simulink model "tracked_robot_alg_loop_converges"  (R2023a)
settings: Solver=FixedStepDiscrete  StartTime=0.0  StopTime=sim_param.t_end  FixedStep=sim_param.dt  RelTol=1e-3  EnableMultiTasking=on
InitFcn:
  | tracked_robot_param
undefined symbols (not defined in the file or in its folder): DiscIntNeverNeededParam, param, path_param, sim_param
libraries: simulink x2
settings Model: PacingRate=0.002500  Creator=david  LastModifiedBy=mfocchi
settings SolverCC: AutoInsertRateTranBlk=on
settings OptimizationCC: DefaultParameterBehavior=Inlined  UseDivisionForNetSlopeComputation=on  GainParamInheritBuiltInType=on  UseFloatMulNetSlope=on  InlineInvariantSignals=on  PassReuseOutputArgsAs=Individual arguments  ZeroExternalMemoryAtStartup=off  ZeroInternalMemoryAtStartup=off  NoFixptDivByZeroProtection=on  EfficientFloat2IntCast=on  LifeSpan=1  OptimizeBlockOrder=speed  DifferentSizesBufferReuse=on  EfficientTunableParamExpr=on
settings DebuggingCC: ParameterTunabilityLossMsg=error  UnderSpecifiedDimensionMsg=warning
settings HardwareCC: ProdLongLongMode=on
settings ModelReferenceCC: ModelReferenceMinAlgLoopOccurrences=on
settings SFSimCC: MATLABDynamicMemAlloc=off
settings RTWCC: Description=Embedded Coder  SystemTargetFile=ert.tlc  TemplateMakefile=ert_default_tmf  TargetLang=C++
settings CodeAppCC: ForceParamTrailComments=on  IgnoreCustomStorageClasses=off  OperatorAnnotations=on  SimulinkDataObjDesc=on  SFDataObjDesc=on  CustomSymbolStrGlobalVar=rt$N$M  CustomSymbolStrType=$N$M  CustomSymbolStrFcn=$N$M$F  CustomSymbolStrMacro=$N$M  InsertBlockDesc=on
settings ERTTargetCC: TargetLangStandard=C++11 (ISO)  GenerateSampleERTMain=on  IncludeMdlTerminateFcn=off  CombineSignalStateStructs=on  CodeInterfacePackaging=C++ class  SupportComplex=off  SupportContinuousTime=on  SupportNonInlinedSFcns=on  SupportVariableSizeSignals=on  InlinedParameterPlacement=NonHierarchical  RootIOFormat=Structure reference  ERTCustomFileTemplate=example_file_process.tlc  ERTFilePackagingFormat=CompactWithDataFile

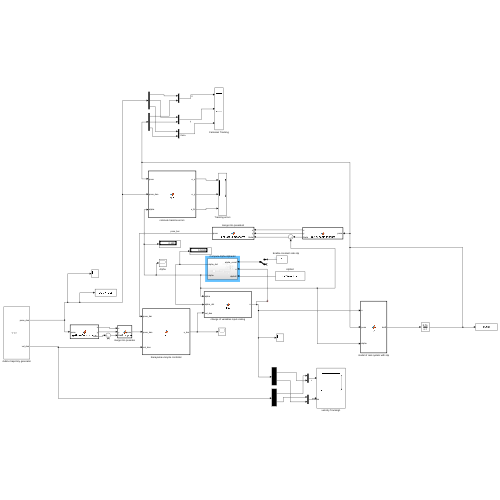
[thumbnail: Simulink's stored preview of the top-level diagram]
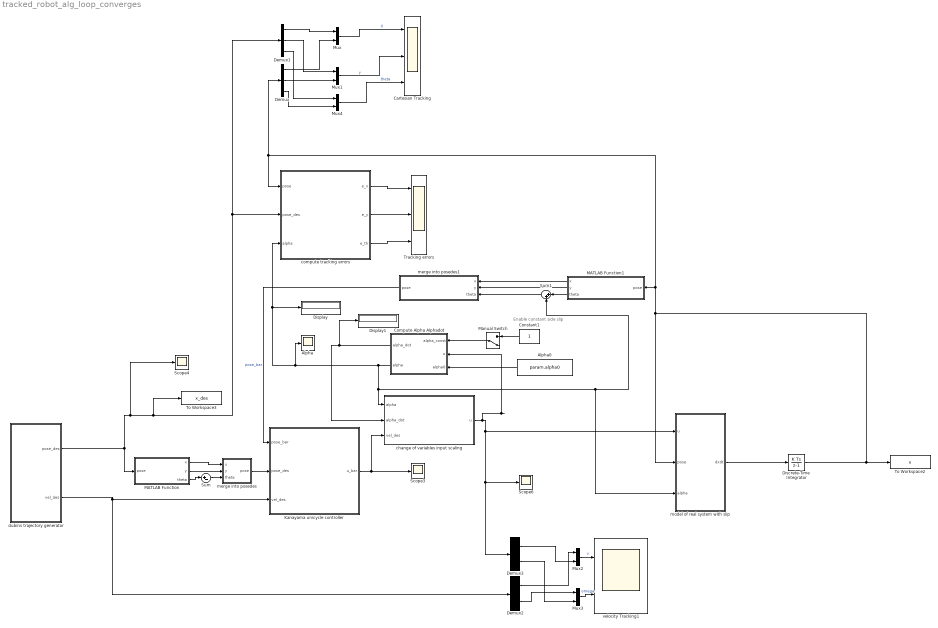
== system tracked_robot_alg_loop_converges ==
  note: Enable constant side slip
  Alpha : Scope
  Alpha0 : Constant  Value=param.alpha0
  Cartesian Tracking : Scope  NumInputPorts=3
  Compute Alpha Alphadot : Subsystem
  Constant1 : Constant
  Demux : Demux  Outputs=3
  Demux1 : Demux  Outputs=3
  Demux2 : Demux  Outputs=2
  Demux3 : Demux  Outputs=2
  Discrete-Time Integrator : DiscreteIntegrator  InitialCondition=sim_param.initial_state  SampleTime=sim_param.dt  ICPrevOutput=DiscIntNeverNeededParam  ICPrevScaledInput=DiscIntNeverNeededParam
  Display : Display
  Display1 : Display
  Kanayama unicycle controller : MATLAB Function  TreatAsAtomicUnit=on
  MATLAB Function : MATLAB Function  TreatAsAtomicUnit=on
  MATLAB Function1 : MATLAB Function  TreatAsAtomicUnit=on
  Manual Switch : ManualSwitch  CurrentSetting=0
  Mux{,1..4} (5 alike) : Mux  Inputs=2
  Scope3 : Scope
  Scope4 : Scope
  Scope6 : Scope
  Sum : Sum  Inputs=|+-
  Sum1 : Sum  Inputs=|++
  To Workspace2 : ToWorkspace  VariableName=x  SaveFormat=Timeseries  SampleTime=-1
      settings: Decimation=sim_param.decimation
  To Workspace3 : ToWorkspace  VariableName=x_des  SaveFormat=Timeseries  SampleTime=-1
      settings: Decimation=sim_param.decimation
  Tracking errors : Scope  NumInputPorts=3
  change of variables input scaling : MATLAB Function  TreatAsAtomicUnit=on
  compute tracking errors : MATLAB Function  TreatAsAtomicUnit=on
  dubins trajectory generator : Subsystem
      mask Display: image('C:\Users\david\Documents\GitHub\tracked_robot_sim\icons\traj_gen.png'); % Use "Edit Image" on toolstrip to change.
  merge into posedes : MATLAB Function  TreatAsAtomicUnit=on
  merge into posedes1 : MATLAB Function  TreatAsAtomicUnit=on
  model of real system with slip : MATLAB Function  TreatAsAtomicUnit=on
  velocity Tracking1 : Scope  NumInputPorts=2
  wires:
  model of real system with slip/1(dxdt) -> Discrete-Time Integrator/1
  dubins trajectory generator/1(pose_des) -> MATLAB Function/1(pose), compute tracking errors/2(pose_des), Demux1/1, To Workspace3/1, Scope4/1
  Discrete-Time Integrator/1 -> To Workspace2/1, MATLAB Function1/1(pose), compute tracking errors/1(pose), Demux/1, model of real system with slip/2(pose)
  Kanayama unicycle controller/1(u_bar) -> Scope3/1, change of variables input scaling/3(vel_des)
  MATLAB Function/1(x) -> merge into posedes/1(x)
  MATLAB Function/2(y) -> merge into posedes/2(y)
  MATLAB Function/3(theta) -> Sum/1
  Sum/1 -> merge into posedes/3(theta)
  merge into posedes/1(pose) -> Kanayama unicycle controller/2(pose_des)
  compute tracking errors/1(e_x) -> Tracking errors/1
  compute tracking errors/2(e_y) -> Tracking errors/2
  compute tracking errors/3(e_th) -> Tracking errors/3
  Alpha0/1 -> Compute Alpha Alphadot/3(alpha0)
  Mux/1 -> Cartesian Tracking/1  "X"
  Mux1/1 -> Cartesian Tracking/2  "y"
  Compute Alpha Alphadot/1(alpha_dot) -> Display1/1, change of variables input scaling/2(alpha_dot)
  Compute Alpha Alphadot/2(alpha) -> change of variables input scaling/1(alpha), Sum1/2, model of real system with slip/3(alpha), Alpha/1, compute tracking errors/3(alpha), Display/1
  Mux2/1 -> velocity Tracking1/1  "v"
  Mux3/1 -> velocity Tracking1/2  "omega"
  dubins trajectory generator/2(vel_des) -> Demux2/1, Kanayama unicycle controller/3(vel_des)
  Demux2/1 -> Mux2/1
  Demux2/2 -> Mux3/1
  Demux3/1 -> Mux2/2
  Demux3/2 -> Mux3/2
  Mux4/1 -> Cartesian Tracking/3  "theta"
  Constant1/1 -> Manual Switch/1
  Manual Switch/1 -> Compute Alpha Alphadot/1(alpha_const)
  MATLAB Function1/1(x) -> merge into posedes1/1(x)
  MATLAB Function1/2(y) -> merge into posedes1/2(y)
  Sum1/1 -> merge into posedes1/3(theta)
  MATLAB Function1/3(theta) -> Sum1/1
  merge into posedes1/1(pose) -> Kanayama unicycle controller/1(pose_bar)  "pose_bar"
  Demux1/1 -> Mux/1
  Demux/1 -> Mux/2
  Demux1/2 -> Mux1/1
  Demux1/3 -> Mux4/1
  Demux/3 -> Mux4/2
  Demux/2 -> Mux1/2
  change of variables input scaling/1(u) -> Compute Alpha Alphadot/2(u), Demux3/1, Scope6/1, model of real system with slip/1(u)

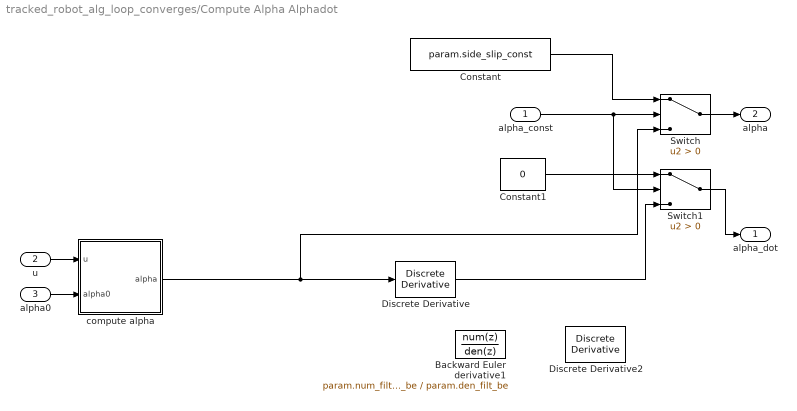
== system tracked_robot_alg_loop_converges/Compute Alpha Alphadot ==
  alpha_const : Inport
  u : Inport  Port=2
  alpha0 : Inport  Port=3
  Backward Euler derivative1 : DiscreteTransferFcn  Numerator=param.num_filt_be  Denominator=param.den_filt_be  InitialStates=1  SampleTime=sim_param.dt
  Constant : Constant  Value=param.side_slip_const
  Constant1 : Constant  Value=0
  Discrete Derivative : simulink/Discrete/Discrete Derivative  gainval=1.0  ICPrevScaledInput=0.0  OutMin=[]  OutMax=[]  OutDataType=fixdt(1, 16)  OutScaling=2^-10  DoSatur=off
  Discrete Derivative2 : simulink/Discrete/Discrete Derivative  gainval=1.0  ICPrevScaledInput=0.0  OutMin=[]  OutMax=[]  OutDataType=fixdt(1, 16)  OutScaling=2^-10  DoSatur=off
  Switch : Switch  Criteria=u2 > Threshold  SaturateOnIntegerOverflow=off  InputSameDT=off
  Switch1 : Switch  Criteria=u2 > Threshold  SaturateOnIntegerOverflow=off  InputSameDT=off
  compute alpha : MATLAB Function  TreatAsAtomicUnit=on
  alpha_dot : Outport
  alpha : Outport  Port=2
  wires:
  alpha0/1 -> compute alpha/2(alpha0)
  u/1 -> compute alpha/1(u)
  compute alpha/1(alpha) -> Discrete Derivative/1, Switch/3
  Constant/1 -> Switch/1
  alpha_const/1 -> Switch1/2, Switch/2
  Constant1/1 -> Switch1/1
  Switch/1 -> alpha/1
  Discrete Derivative/1 -> Switch1/3
  Switch1/1 -> alpha_dot/1

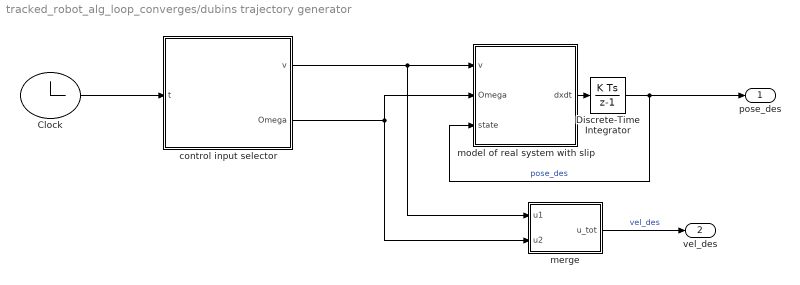
== system tracked_robot_alg_loop_converges/dubins trajectory generator ==
  Clock : Clock
  Discrete-Time Integrator : DiscreteIntegrator  InitialCondition=path_param.init_pose  SampleTime=sim_param.dt  ICPrevOutput=DiscIntNeverNeededParam  ICPrevScaledInput=DiscIntNeverNeededParam
  control input selector : MATLAB Function  TreatAsAtomicUnit=on
  merge : MATLAB Function  TreatAsAtomicUnit=on
  model of real system with slip : MATLAB Function  TreatAsAtomicUnit=on
  pose_des : Outport
  vel_des : Outport  Port=2
  wires:
  Discrete-Time Integrator/1 -> pose_des/1, model of real system with slip/3(state)  "pose_des"
  merge/1(u_tot) -> vel_des/1  "vel_des"
  control input selector/1(v) -> merge/1(u1), model of real system with slip/1(v)
  control input selector/2(Omega) -> model of real system with slip/2(Omega), merge/2(u2)
  Clock/1 -> control input selector/1(t)
  model of real system with slip/1(dxdt) -> Discrete-Time Integrator/1

== matlab function tracked_robot_alg_loop_converges/dubins trajectory generator/model of real system with slip ==
  data: v input; Omega input; dxdt output; state input
function dxdt = fcn(v, Omega, state)

    theta = state(3);
    
    dxdt = [v*cos(theta) , v*sin(theta), Omega];
end

== matlab function tracked_robot_alg_loop_converges/Compute Alpha Alphadot/compute alpha ==
  data: u input size=2; alpha0 input size=1; alpha output size=1
function alpha = fcn(u, alpha0)
    v = u(1);
    omega = u(2);
    %alpha = alpha0*omega^2/((v+0.0001)^2);
    if (abs(v) < 0.001)
        alpha = 0;
    else 
        alpha = alpha0*omega^2/((v+0.0001)^2);
    end

end

== matlab function tracked_robot_alg_loop_converges/MATLAB Function1 ==
  data: x output; pose input; y output; theta output
function [x,y,theta] = getPoseComponents(pose)
x = pose(1);
y = pose(2);
theta = pose(3);

== matlab function tracked_robot_alg_loop_converges/merge into posedes1 ==
  data: pose output; x input; y input; theta input
function pose = getPoseComponents(x,y,theta)
pose = [x,y,theta];

== matlab function tracked_robot_alg_loop_converges/dubins trajectory generator/control input selector ==
  data: t input; v output double size=1; Omega output double size=1; path_param parameter
function [v,Omega] = fcn(t, path_param)
    % select the right control input in function of the current time. In
    % the params 5 vectors must be defined:
    % time_vec : list of n times [t1... tn]
    % 

    idx = find(t >= path_param.time_vec, 1, 'last');
    idx = idx(1);
    if(idx >= length(path_param.linear_velocity.q))
        idx = length(path_param.linear_velocity.q);
    end
    vq = path_param.linear_velocity.q(idx);
    vm = path_param.linear_velocity.m(idx);
    aq = path_param.angular_velocity.q(idx);
    am =  path_param.angular_velocity.m(idx);
    
    v     = vm*t + vq;
    Omega = am*t + aq;
end

== matlab function tracked_robot_alg_loop_converges/model of real system with slip ==
  data: u input; dxdt output; pose input; alpha input
function dxdt = fcn(u, pose, alpha)

theta = pose(3);

v     = u(1);
Omega = u(2);

dxdt = [v*cos(theta + alpha) / cos(alpha), v*sin(theta + alpha) / cos(alpha), Omega];

== matlab function tracked_robot_alg_loop_converges/Kanayama unicycle controller ==
  data: pose_bar input; pose_des input; u_bar output size=[1,2]; vel_des input; ctrl_param parameter
function u_bar = fcn(pose_bar, pose_des, vel_des, ctrl_param)
    % compute the control for a unicycle using Lyapunov theory
    u_bar = zeros(1,2);

    theta_des = pose_des(3);
    theta_bar = pose_bar(3);

 
 
    if ctrl_param.controller_type == 1

        error_x     = pose_bar(1) - pose_des(1);
        error_y     = pose_bar(2) - pose_des(2);
        error_theta = theta_bar - theta_des;

        V_hat = vel_des(1);
        Omega_hat = vel_des(2);
    
        Kp = ctrl_param.Kp;
        K_theta = ctrl_param.K_theta;
    
        psi = atan2(error_y, error_x);
        alpha = (theta_bar + theta_des) / 2.0;
        error_xy = sqrt(error_x^2 + error_y^2);
    
    
        dv = - Kp * error_xy * cos(theta_bar - psi);
        domega =  - K_theta * error_theta - V_hat * sinc(error_theta / (2)) * error_xy * sin(psi - alpha);
    
        u_bar(1) = V_hat + dv;
        u_bar(2) = Omega_hat + domega;
    
    
    
    elseif ctrl_param.controller_type == 2
    
        error_x     = pose_des(1) - pose_bar(1);
        error_y     = pose_des(2) - pose_bar(2);
        error_theta = theta_des - theta_bar;
        % Kanayama controller (not polar variables) we consider both ex and ey
        % separately!
        V_d= vel_des(1);
        Omega_d = vel_des(2);
    
        Kx = ctrl_param.Kp;
        K_theta = ctrl_param.K_theta;
    
        %express errors in the base frame
        base_error_x     = cos(theta_bar) * error_x + sin(theta_bar)*error_y;
        base_error_y     = -sin(theta_bar) *error_x + cos(theta_bar)*error_y;
    
        %command velocity
        u_bar(1) = V_d*cos(error_theta) + Kx*base_error_x;
        u_bar(2) = Omega_d + K_theta*sin(error_theta) + V_d*base_error_y;
    
    else
        disp('wrong controller')
    end



end

== matlab function tracked_robot_alg_loop_converges/merge into posedes ==
  data: pose output; x input; y input; theta input
function pose = getPoseComponents(x,y,theta)
pose = [x,y,theta];

== matlab function tracked_robot_alg_loop_converges/MATLAB Function ==
  data: x output; pose input; y output; theta output
function [x,y,theta] = getPoseComponents(pose)
x = pose(1);
y = pose(2);
theta = pose(3);

== matlab function tracked_robot_alg_loop_converges/change of variables input scaling ==
  data: alpha input; alpha_dot input; u output size=[1,2]; vel_des input
function u = fcn(alpha, alpha_dot,vel_des)
    u = zeros(1,2);

    v_bar = vel_des(1);
    Omega_bar = vel_des(2);
    
    u(1) = v_bar * cos(alpha); 
    u(2) = Omega_bar - alpha_dot; 

end

== matlab function tracked_robot_alg_loop_converges/dubins trajectory generator/merge ==
  data: u1 input; u_tot output; u2 input
function u_tot = fcn(u1,u2)
    u_tot = [u1,u2];
end

== matlab function tracked_robot_alg_loop_converges/compute tracking errors ==
  data: pose input; pose_des input; alpha input; e_x output; e_y output; e_th output
function [e_x,e_y, e_th] = fcn(pose, pose_des, alpha)
    % compute the tracking errors with respect to the reference input. Note that the
    % orientation error is not the one of the robot but takes into account
    % the side slip angle.

    theta_des = pose_des(3);
    theta = pose(3);

    e_x = pose(1)-pose_des(1);
    e_y = pose(2)-pose_des(2);
    e_th = (theta+alpha)  - theta_des; % whenever the compensation does its job theta_bar converges to theta+alpha so we need to check if theta+alpha converges to theta_des
                                       % if you want theta converging to
                                       % correct orient then you need to
                                       % add an offset to theta des
                                       
end
